simulink model "LQR_NLE"  (R2024b)
settings: Solver=VariableStepAuto  StartTime=0.0  StopTime=10.0  RelTol=1e-3
values from neighbouring files (symbols this model uses):
  disorder_times = [10, 14]    [assignment1.m]
  lqr_stop_time = 15    [assignment1.m]
  u_control = 0.5    [assignment1.m]
  z = 0.1    [assignment1.m]
undefined symbols (not defined in the file or in its folder): K, N
settings Model: Creator=lukiq  LastModifiedBy=lukiq
settings DebuggingCC: AlgebraicLoopMsg=none

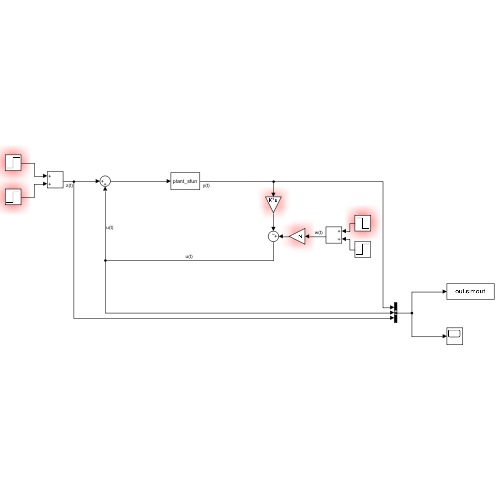
[thumbnail: Simulink's stored preview of the top-level diagram]
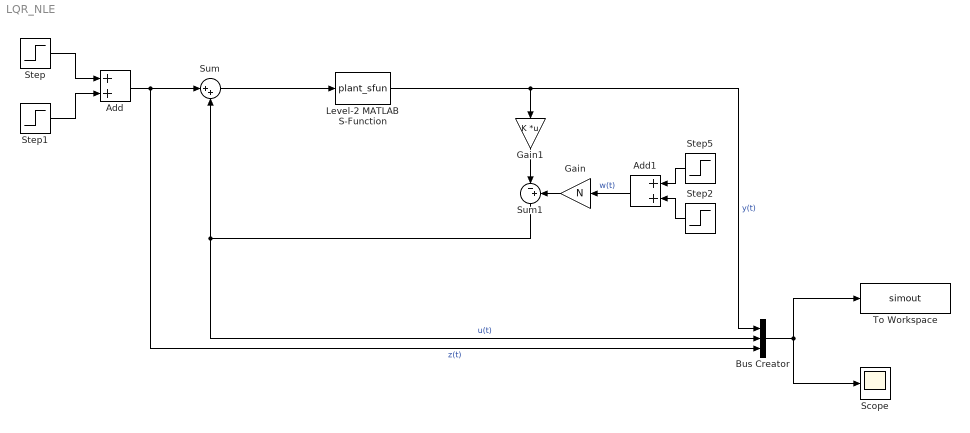
== system LQR_NLE ==
  Add : Sum
  Add1 : Sum
  Bus Creator : BusCreator  Inputs=3
  Gain : Gain  Gain=N
  Gain1 : Gain  Gain=K  Multiplication=Matrix(K*u)
  Level-2 MATLAB S-Function : M-S-Function  FunctionName=plant_sfun  Parameters=odeHandleSimulink, p, u, outIdx
  Scope : Scope
  Step : Step  Time=disorder_times(1)  After=- z * u_control  SampleTime=0
  Step1 : Step  Time=disorder_times(2)  After=z * u_control  SampleTime=0
  Step2 : Step  SampleTime=0
  Step5 : Step  Time=lqr_stop_time  After=-1  SampleTime=0
  Sum : Sum  Inputs=|++
  Sum1 : Sum  Inputs=|-+
  To Workspace : ToWorkspace  VariableName=simout  SaveFormat=Timeseries  SampleTime=-1
  wires:
  Sum/1 -> Level-2 MATLAB S-Function/1
  Sum1/1 -> Bus Creator/2, Sum/2  "u(t)"
  Add/1 -> Sum/1, Bus Creator/3  "z(t)"
  Step/1 -> Add/1
  Step1/1 -> Add/2
  Bus Creator/1 -> Scope/1, To Workspace/1
  Gain/1 -> Sum1/2
  Gain1/1 -> Sum1/1
  Step2/1 -> Add1/2
  Step5/1 -> Add1/1
  Add1/1 -> Gain/1  "w(t)"
  Level-2 MATLAB S-Function/1 -> Bus Creator/1, Gain1/1  "y(t)"
